simulink model "Test_Encoder_8_to_3"  (Simulink 8.1)
settings: Solver=ode45  StartTime=0.0  StopTime=len  RelTol=1e-3
libraries: commutil2 x2, Encoders_Lib x1
settings Model: Creator=N  LastModifiedBy=uzivatel
settings DataIOCC: LimitDataPoints=off  SignalLoggingSaveFormat=Dataset
settings OptimizationCC: ExpressionDepthLimit=128
settings DebuggingCC: UnderspecifiedInitializationDetection=Simplified  MergeDetectMultiDrivingBlocksExec=error  SolverPrmCheckMsg=none  FcnCallInpInsideContextMsg=EnableAllAsError  FrameProcessingCompatibilityMsg=error  StateNameClashWarn=none
settings HardwareCC: ProdBitPerPointer=64  ProdLargestAtomicFloat=Float  ProdIntDivRoundTo=Zero  ProdEndianess=LittleEndian  ProdHWDeviceType=Intel->x86-64 (Windows64)
settings ModelReferenceCC: PropagateSignalLabelsOutOfModel=on
settings GRTTargetCC: CodeReplacementLibrary=None  CombineOutputUpdateFcns=on  CPPClassGenCompliant=on  GRTInterface=off

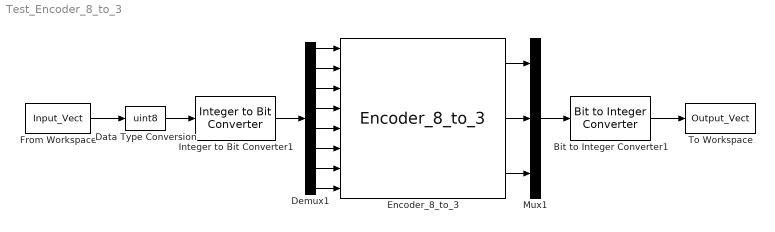
== system Test_Encoder_8_to_3 ==
  Bit to Integer Converter1 : commutil2/Bit to Integer Converter  nbits=3  bitOrder=LSB first  signedOutputValues=Unsigned  outDtype=uint8  outDtypeSigned=Inherit via internal rule
  Data Type Conversion : DataTypeConversion  OutDataTypeStr=uint8
  Demux1 : Demux  Outputs=8
  Encoder_8_to_3 : Encoders_Lib/Encoders_Lib/Encoder_8_to_3
  From Workspace : FromWorkspace  VariableName=Input_Vect  SampleTime=1  Interpolate=off  OutputAfterFinalValue=Holding final value
  Integer to Bit Converter1 : commutil2/Integer to Bit Converter  nbits=8  signedInputValues=Unsigned  bitOrder=LSB first  outDtype=boolean
  Mux1 : Mux  Inputs=3
  To Workspace : ToWorkspace  VariableName=Output_Vect  SampleTime=1
  wires:
  Integer to Bit Converter1/1 -> Demux1/1
  Demux1/1 -> Encoder_8_to_3/1
  Demux1/2 -> Encoder_8_to_3/2
  Demux1/3 -> Encoder_8_to_3/3
  Demux1/4 -> Encoder_8_to_3/4
  Demux1/5 -> Encoder_8_to_3/5
  Demux1/6 -> Encoder_8_to_3/6
  Demux1/7 -> Encoder_8_to_3/7
  Demux1/8 -> Encoder_8_to_3/8
  Mux1/1 -> Bit to Integer Converter1/1
  Encoder_8_to_3/2 -> Mux1/2
  Encoder_8_to_3/1 -> Mux1/1
  Encoder_8_to_3/3 -> Mux1/3
  Data Type Conversion/1 -> Integer to Bit Converter1/1
  Bit to Integer Converter1/1 -> To Workspace/1
  From Workspace/1 -> Data Type Conversion/1
